simulink model "cruise_control"  (R2021b)
settings: Solver=FixedStepAuto  StartTime=0.0  StopTime=50  RelTol=1e-3
PreLoadFcn:
  | clearvars;
  | m = 1000;
  | b = 50;
  | Ts = 0.01;
  | u = 100;
  | Kp = 800;
  | Ki = 100;
  | Kd = 0;
settings Model: Creator=adish  LastModifiedBy=adish
settings OptimizationCC: UseDivisionForNetSlopeComputation=on

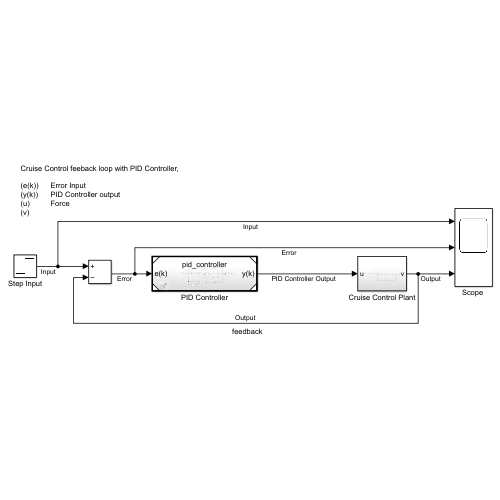
[thumbnail: Simulink's stored preview of the top-level diagram]
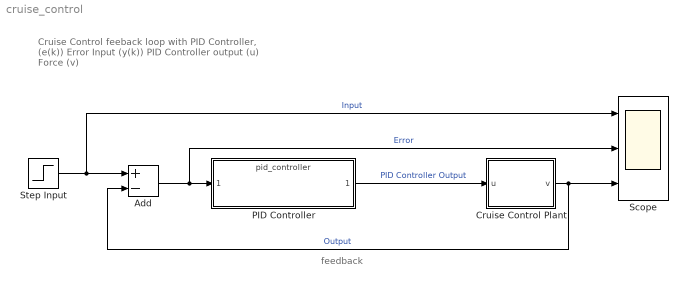
== system cruise_control ==
  note: Cruise Control feeback loop with PID Controller,
      |
      | (e(k))	Error Input
      | (y(k))	PID Controller output
      | (u)		Force
      | (v)
  note: feedback
  Add : Sum  Inputs=+-
  Cruise Control Plant : Subsystem
  PID Controller : ModelReference  ModelNameDialog=pid_controller.slx  SimulationMode=Normal  ModelReferenceVersion=1.83
  "Scope " : Scope  NumInputPorts=3
  Step Input : Step  After=100  SampleTime=0.01
  wires:
  Step Input/1 -> "Scope "/1, Add/1  "Input"
  Cruise Control Plant/1(v) -> "Scope "/3, Add/2  "Output"
  Add/1 -> PID Controller/1, "Scope "/2  "Error"
  PID Controller/1 -> Cruise Control Plant/1(u)  "PID Controller Output"

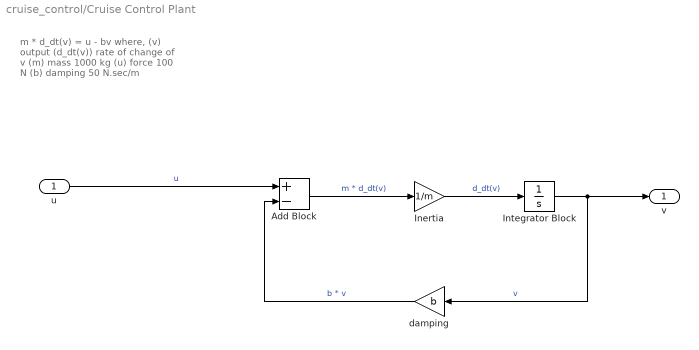
== system cruise_control/Cruise Control Plant ==
  note: m * d_dt(v) = u - bv
      | where,
      | (v)	output
      | (d_dt(v))		rate of change of v
      | (m)	mass	1000 kg
      | (u)	force		100 N
      | (b)	damping		50 N.sec/m
  u : Inport
  Add Block : Sum  Inputs=+-
  Inertia : Gain  Gain=1/m
  "Integrator Block " : Integrator
  damping : Gain  Gain=b
  v : Outport
  wires:
  Add Block/1 -> Inertia/1  "m * d_dt(v)"
  damping/1 -> Add Block/2  "b * v"
  Inertia/1 -> "Integrator Block "/1  "d_dt(v)"
  "Integrator Block "/1 -> v/1, damping/1  "v"
  u/1 -> Add Block/1  "u"
